simulink subsystem "Volume_flow_with_processing"  (R2025b)
settings: Solver=VariableStepAuto  StartTime=0.0  StopTime=10.0  RelTol=1e-3
model mask{InitialCondition=100, Max_cap=10, Diameter=24.5}
  mask prompts: InitialCondition "Initial level:"; Max_cap "Max capacity"
settings Model: Creator=Soere  LastModifiedBy=klump

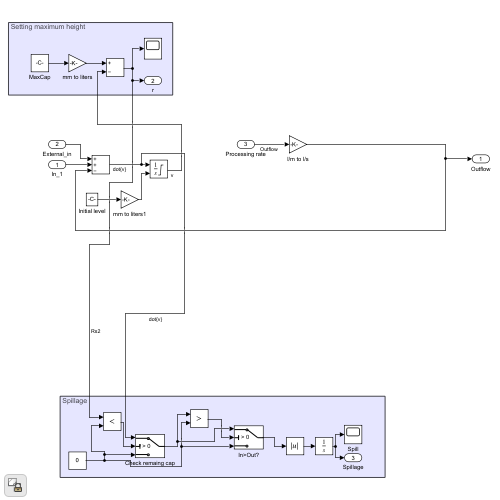
[thumbnail: Simulink's stored preview of the top-level diagram]
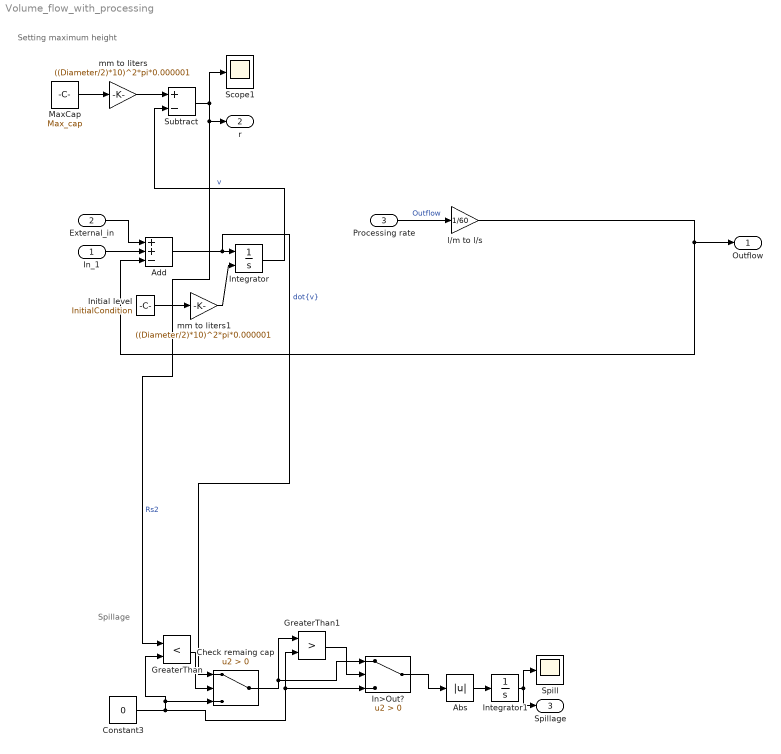
== system Volume_flow_with_processing ==
  note: Setting maximum height
  note: Spillage
  In_1 : Inport
  External_in : Inport  Port=2
  Processing rate : Inport  Port=3  OutMin=0  OutMax=100
  Abs : Abs  SaturateOnIntegerOverflow=off
  Add : Sum  Inputs=++-
  Check remaing cap : Switch  Criteria=u2 > Threshold  SaturateOnIntegerOverflow=off  InputSameDT=off
  Constant3 : Constant  Value=0
  GreaterThan : RelationalOperator  Operator=<  OutDataTypeStr=boolean  RndMeth=Simplest  InputSameDT=off
  GreaterThan1 : RelationalOperator  Operator=>  OutDataTypeStr=boolean  RndMeth=Simplest  InputSameDT=off
  In>Out? : Switch  Criteria=u2 > Threshold  SaturateOnIntegerOverflow=off  InputSameDT=off
  Initial level : Constant  Value=InitialCondition
  Integrator : Integrator  InitialConditionSource=external  InitialCondition=100  LimitOutput=on  UpperSaturationLimit=Max_cap  LowerSaturationLimit=0
  Integrator1 : Integrator
  MaxCap : Constant  Value=Max_cap
  Scope1 : Scope
      settings: ActiveDisplayYMinimum=-16.555361778066185  ActiveDisplayYMaximum=118.63213822193381  DataLoggingVariableName=ScopeData21
  Spill : Scope
      settings: ActiveDisplayYMinimum=-1.8046784978438728  ActiveDisplayYMaximum=16.24210648059486  DataLoggingVariableName=ScopeData74
  Subtract : Sum  Inputs=+-
  l/m to l/s : Gain  Gain=1/60
  mm to liters : Gain  Gain=((Diameter/2)*10)^2*pi*0.000001
  mm to liters1 : Gain  Gain=((Diameter/2)*10)^2*pi*0.000001
  Outflow : Outport
  r : Outport  Port=2
  Spillage : Outport  Port=3
  wires:
  l/m to l/s/1 -> Outflow/1, Add/3
  mm to liters1/1 -> Integrator/2
  Initial level/1 -> mm to liters1/1
  mm to liters/1 -> Subtract/1
  MaxCap/1 -> mm to liters/1
  External_in/1 -> Add/1
  In_1/1 -> Add/2
  Integrator/1 -> Subtract/2  "v"
  Processing rate/1 -> l/m to l/s/1  "Outflow"
  Check remaing cap/1 -> GreaterThan1/1, In>Out?/1
  Subtract/1 -> Scope1/1, r/1, GreaterThan/1  "Rs2"
  Abs/1 -> Integrator1/1
  Constant3/1 -> GreaterThan/2, Check remaing cap/3, GreaterThan1/2, In>Out?/3
  Integrator1/1 -> Spillage/1, Spill/1
  Add/1 -> Integrator/1, Check remaing cap/1  "dot{v}"
  In>Out?/1 -> Abs/1
  GreaterThan/1 -> Check remaing cap/2
  GreaterThan1/1 -> In>Out?/2
